simulink library "INT_Gbx_Data"  (R2016b)
settings: Solver=VariableStepAuto  StartTime=0.0  StopTime=10.0  RelTol=1e-3
settings Model: Creator=bianxuyin  LastModifiedBy=bianxuyin

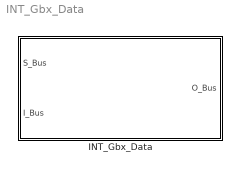
== system INT_Gbx_Data ==
  INT_Gbx_Data : Subsystem

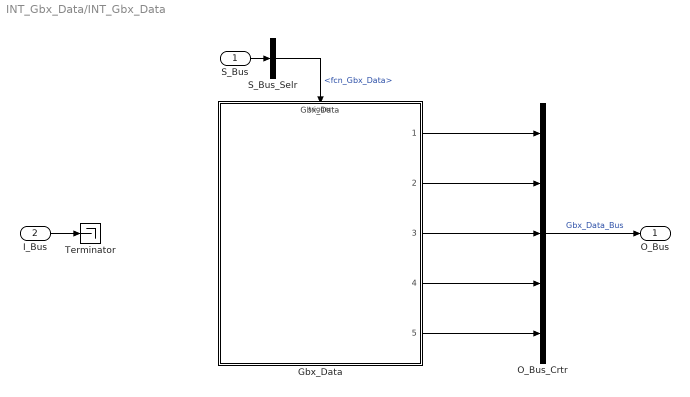
== system INT_Gbx_Data/INT_Gbx_Data ==
  S_Bus : Inport
  I_Bus : Inport  Port=2
  Gbx_Data : ModelReference  ModelNameDialog=Gbx_Data  SimulationMode=Normal  ModelReferenceVersion=1.5  TriggerPortName=function  TriggerPortTriggerType=function-call  TriggerPortStatesWhenEnabling=held
  O_Bus_Crtr : BusCreator  Inputs=5
  S_Bus_Selr : BusSelector  OutputSignals=fcn_Gbx_Data
  Terminator : Terminator
  O_Bus : Outport
  wires:
  S_Bus_Selr/1 -> Gbx_Data/Trigger  "<fcn_Gbx_Data>"
  S_Bus/1 -> S_Bus_Selr/1
  I_Bus/1 -> Terminator/1
  O_Bus_Crtr/1 -> O_Bus/1  "Gbx_Data_Bus"
  Gbx_Data/1 -> O_Bus_Crtr/1
  Gbx_Data/2 -> O_Bus_Crtr/2
  Gbx_Data/3 -> O_Bus_Crtr/3
  Gbx_Data/4 -> O_Bus_Crtr/4
  Gbx_Data/5 -> O_Bus_Crtr/5
